simulink model "turbofan"  (R2012b)
settings: Solver=FixedStepDiscrete  StartTime=0.0  StopTime=10.5  FixedStep=0.015  RelTol=1e-3
libraries: Lib_Turbo_Shaft_TMATS x2, Lib_Solve_SSNRSolverJC_TMATS x1
settings Model: Creator=tlavelle  LastModifiedBy=tlavelle

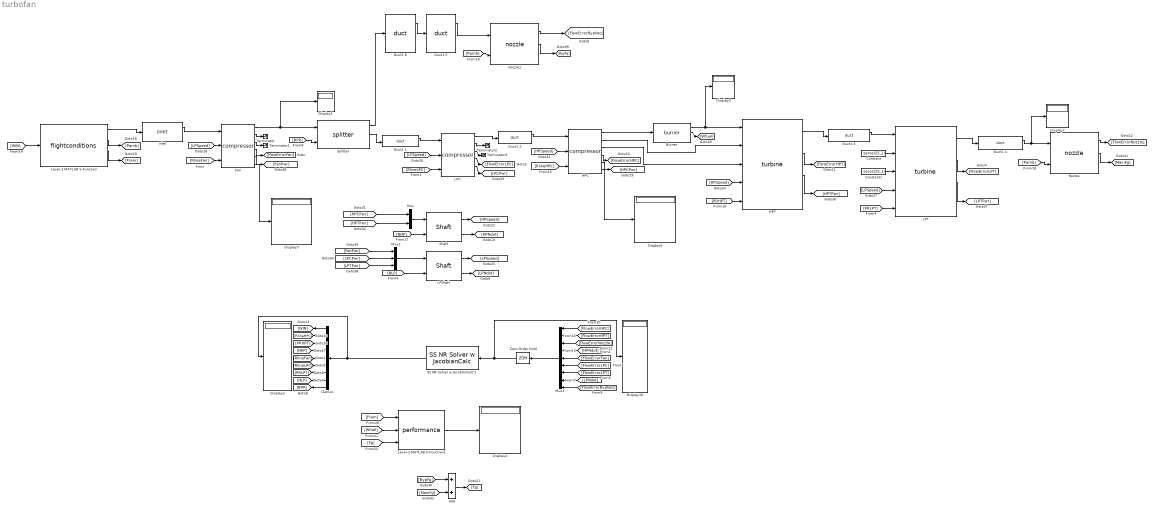
== system turbofan ==
  Add : Sum
  "Burner " : M-S-Function  FunctionName=burner  Parameters=Wfuel,hFuel,dP  mask{Wfuel=.0187, hFuel=-1200, dP=.055}
      mask prompts: Wfuel "FAR"; hFuel "Fuel enthalpy"
      mask Display:
      | color('blue'); port_label('input',1,'Flow In')
      | color('blue'); port_label('output',1,'Flow Out')
      | 
      | color('black'); port_label('output',2,'Wfuel')
  Constant : Constant  Value=zeros(25,1)
  Constant1 : Constant  Value=zeros(25,1)
  Demux : Demux  Outputs=9
  Display{1..7,16} (8 alike) : Display
  Duct1 1 : M-S-Function  FunctionName=duct  Parameters=dP  mask{dP=.0025}
      mask Display:
      | color('blue'); port_label('input',1,'Flow In')
      | color('blue'); port_label('output',1,'Flow Out')
  Duct1 2 : M-S-Function  FunctionName=duct  Parameters=dP  mask{dP=.0025}
      mask Display:
      | color('red'); port_label('input',1,'Flow In')
      | color('red'); port_label('output',1,'Flow Out')
  Duct1 3 : M-S-Function  FunctionName=duct  Parameters=dP  mask{dP=.005}
      mask Display:
      | color('blue'); port_label('input',1,'Flow In')
      | color('blue'); port_label('output',1,'Flow Out')
  Duct1 4 : M-S-Function  FunctionName=duct  Parameters=dP  mask{dP=.01}
      mask Display:
      | color('blue'); port_label('input',1,'Flow In')
      | color('blue'); port_label('output',1,'Flow Out')
  Duct1 5 : M-S-Function  FunctionName=duct  Parameters=dP  mask{dP=.0075}
      mask Display:
      | color('blue'); port_label('input',1,'Flow In')
      | color('blue'); port_label('output',1,'Flow Out')
  Duct1 6 : M-S-Function  FunctionName=duct  Parameters=dP  mask{dP=.0025}
      mask Display:
      | color('blue'); port_label('input',1,'Flow In')
      | color('blue'); port_label('output',1,'Flow Out')
  Fan : M-S-Function  FunctionName=compressor  Parameters=MapFile,NcDes,effDes,PRdes,RlineDes,Wfrac1,hfrac1,Pfrac1,Wfrac2,hfrac2,Pfrac2,s_eff_in,s_PR_in,s_Wc_in,s_C_Nc_in,IDes  mask{MapFile='FAN.map', NcDes=100, effDes=.867, PRdes=1.645, RlineDes=2.3706, Wfrac1=0, hfrac1=0, Pfrac1=0, Wfrac2=0, hfrac2=0, Pfrac2=0, s_eff_in=0, s_PR_in=0, s_Wc_in=0, s_C_Nc_in=0, IDes=0}
      mask prompts: Wfrac1 "Weight Flow Fraction Bleed1"; hfrac1 "Enthalpy Fraction Bleed 1"; Pfrac1 "Pressure Fraction Bleed 1"; Wfrac2 "Weight Flow Fraction Bleed2"; hfrac2 "Enthalpy Fraction Bleed 2"; Pfrac2 "Pressure Fraction 2"; s_eff_in "Efficiency map scalar"; s_PR_in "Pressure ratio map scalar"; s_Wc_in "Corrected weight flow map scalar"; s_C_Nc_in "Corrected speed map scalar"
      mask Display:
      | color('blue'); port_label('input',1,'Flow In')
      | color('red'); port_label('input',2,'Speed')
      | color('darkgreen'); port_label('input',3,'Rline')
      | 
      | color('blue'); port_label('output',1,'Flow Out')
      | color('blue'); port_label('output',2,'Bleed 1')
      | color('blue'); port_label('output',3,'Bleed 2')
      | color('green'); port_label('output',4,'Flow Error')
      | color('black'); port_label('output',5,'Power')
  HPC : M-S-Function  FunctionName=compressor  Parameters=MapFile,NcDes,effDes,PRdes,RlineDes,Wfrac1,hfrac1,Pfrac1,Wfrac2,hfrac2,Pfrac2,s_eff_in,s_PR_in,s_Wc_in,s_C_Nc_in,IDes  mask{MapFile='HPC.map', NcDes=100, effDes=.865, PRdes=5.609, RlineDes=2.0424, Wfrac1=.055, hfrac1=1, Pfrac1=1, Wfrac2=.035, hfrac2=1., Pfrac2=1., s_eff_in=0, s_PR_in=0, s_Wc_in=0, s_C_Nc_in=0, IDes=0}
      mask prompts: Wfrac1 "Weight Flow Fraction Bleed1"; hfrac1 "Enthalpy Fraction Bleed 1"; Pfrac1 "Pressure Fraction Bleed 1"; Wfrac2 "Weight Flow Fraction Bleed2"; hfrac2 "Enthalpy Fraction Bleed 2"; Pfrac2 "Pressure Fraction 2"; s_eff_in "Efficiency map scalar"; s_PR_in "Pressure ratio map scalar"; s_Wc_in "Corrected weight flow map scalar"; s_C_Nc_in "Corrected speed map scalar"
      mask Display:
      | color('blue'); port_label('input',1,'Flow In')
      | color('red'); port_label('input',2,'Speed')
      | color('darkgreen'); port_label('input',3,'Rline')
      | 
      | color('blue'); port_label('output',1,'Flow Out')
      | color('blue'); port_label('output',2,'Bleed 1')
      | color('blue'); port_label('output',3,'Bleed 2')
      | color('green'); port_label('output',4,'Flow Error')
      | color('black'); port_label('output',5,'Power')
  HPT : M-S-Function  FunctionName=turbine  Parameters=MapFile,NcDes,effDes,PRmapDes,Ndes,BSW1,BSW2,s_eff,s_Wc,s_C_Nc,s_PR,IDes  mask{MapFile='HPT1.map', NcDes=100, effDes=.913, PRmapDes=4.9299, Ndes=7499, BSW1=1, BSW2=0, s_eff=0, s_Wc=0, s_C_Nc=0, s_PR=0, IDes=0}
      mask prompts: MapFile "Map File"; NcDes "Design Speed"; effDes "Design efficiency"; PRmapDes "Design Pressure Ratio Map"; Ndes "N des"; BSW1 "Bleed 1 Switch (1 front 0 back)"; BSW2 "Bleed 2 Swtich (1 front 0 back )"; s_eff "Input map efficiency scalar"; s_Wc "Input map correct weight flow scala"; s_C_Nc "Input map speed scalar"; s_PR "Input map pressure ratio scalar"
      mask Display:
      | color('blue'); port_label('input',1,'Flow In')
      | color('blue'); port_label('input',2,'Bleed 1')
      | color('blue'); port_label('input',3,'Bleed 2')
      | color('red'); port_label('input',4,'Speed')
      | color('darkgreen'); port_label('input',5,'PR')
      | 
      | color('blue'); port_label('output',1,'Flow Out')
      | color('green'); port_label('output',2,'Flow Error')
      | color('black'); port_label('output',3,'Power')
  Inlet : M-S-Function  FunctionName=inlet  Parameters=recovery  mask{recovery=.995}
      mask Display:
      | color('blue'); port_label('input',1,'Flow In')
      | color('blue'); port_label('output',1,'Flow Out')
  LPC : M-S-Function  FunctionName=compressor  Parameters=MapFile,NcDes,effDes,PRdes,RlineDes,Wfrac1,hfrac1,Pfrac1,Wfrac2,hfrac2,Pfrac2,s_eff_in,s_PR_in,s_Wc_in,s_C_Nc_in,IDes  mask{MapFile='LPC.map', NcDes=100, effDes=.868, PRdes=2.488, RlineDes=1.7664, Wfrac1=0, hfrac1=0, Pfrac1=0, Wfrac2=0, hfrac2=0, Pfrac2=0, s_eff_in=0, s_PR_in=0, s_Wc_in=0, s_C_Nc_in=0, IDes=0}
      mask prompts: Wfrac1 "Weight Flow Fraction Bleed1"; hfrac1 "Enthalpy Fraction Bleed 1"; Pfrac1 "Pressure Fraction Bleed 1"; Wfrac2 "Weight Flow Fraction Bleed2"; hfrac2 "Enthalpy Fraction Bleed 2"; Pfrac2 "Pressure Fraction 2"; s_eff_in "Efficiency map scalar"; s_PR_in "Pressure ratio map scalar"; s_Wc_in "Corrected weight flow map scalar"
      mask Display:
      | color('blue'); port_label('input',1,'Flow In')
      | color('red'); port_label('input',2,'Speed')
      | color('darkgreen'); port_label('input',3,'Rline')
      | 
      | color('blue'); port_label('output',1,'Flow Out')
      | color('blue'); port_label('output',2,'Bleed 1')
      | color('blue'); port_label('output',3,'Bleed 2')
      | color('green'); port_label('output',4,'Flow Error')
      | color('black'); port_label('output',5,'Power')
  LPShaft : Lib_Turbo_Shaft_TMATS/Shaft  Shaft_Inertia_M=1000
  LPT : M-S-Function  FunctionName=turbine  Parameters=MapFile,NcDes,effDes,PRmapDes,Ndes,BSW1,BSW2,s_eff,s_Wc,s_C_Nc,s_PR,IDes  mask{MapFile='LPT.map', NcDes=100, effDes=.93, PRmapDes=6.4203, Ndes=3723, BSW1=1, BSW2=1, s_eff=0, s_Wc=0, s_C_Nc=0, s_PR=0, IDes=0}
      mask prompts: MapFile "Map File"; NcDes "Design Speed"; effDes "Design efficiency"; PRmapDes "Design Pressure Ratio Map"; Ndes "N des"; BSW1 "Bleed 1 Switch (1 front 0 back)"; BSW2 "Bleed 1 Switch (1 front 0 back)"; s_eff "Input map efficiency scalar"; s_Wc "Input map correct weight flow scalar"; s_C_Nc "Input map speed scalar"; s_PR "Input map pressure ratio scalar"
      mask Display:
      | color('blue'); port_label('input',1,'Flow In')
      | color('blue'); port_label('input',2,'Bleed 1')
      | color('blue'); port_label('input',3,'Bleed 2')
      | color('red'); port_label('input',4,'Speed')
      | color('darkgreen'); port_label('input',5,'PR')
      | 
      | color('blue'); port_label('output',1,'Flow Out')
      | color('green'); port_label('output',2,'Flow Error')
      | color('black'); port_label('output',3,'Power')
  Level-2 MATLAB S-Function : M-S-Function  FunctionName=flightconditions  Parameters=alt,MN,dTs  mask{alt=34000, MN=.8, dTs=0}
      mask prompts: alt "altitude"; MN "Mach Number"; dTs "Ambient Temperature Delta"
      mask Display:
      | color('darkgreen'); port_label('input',1,'Weight Flow')
      | 
      | color('blue'); port_label('output',1,'Flow Out')
      | color('black'); port_label('output',2,'Ambient Pressure')
      | color('black'); port_label('output',3,'Fram')
  Level-2 MATLAB S-Function1 : M-S-Function  FunctionName=performance
      mask Display:
      | color('black'); port_label('input',1,'Fram')
      | color('black'); port_label('input',2,'Wfuel')
      | color('black'); port_label('input',3,'Fg')
      | 
      | color('black'); port_label('output',1,'Performance')
  Mux : Mux  Inputs=2
  Mux1 : Mux  Inputs=9
  Mux2 : Mux  Inputs=3
  Nozzle : M-S-Function  FunctionName=nozzle  Parameters=Wdes,Cfg,Ath_in,IDes  mask{Wdes=113.51, Cfg=.9978, Ath_in=0, IDes=0}
      mask prompts: Wdes "Design Flow"; Ath_in "Throat input area"
      mask Display:
      | color('blue'); port_label('input',1,'Flow In')
      | color('black'); port_label('input',2,'Ambient Pressure')
      | 
      | color('green'); port_label('output',1,'Flow Error')
      | color('black'); port_label('output',2,'Fg')
  Nozzle1 : M-S-Function  FunctionName=nozzle  Parameters=Wdes,Cfg,Ath_in,IDes  mask{Wdes=562.61, Cfg=.9978, Ath_in=0, IDes=0}
      mask prompts: Wdes "Design Flow"; Ath_in "Throat area input"
      mask Display:
      | color('blue'); port_label('input',1,'Flow In')
      | color('black'); port_label('input',2,'Ambient Pressure')
      | 
      | color('green'); port_label('output',1,'Flow Error')
      | color('black'); port_label('output',2,'Fg')
  SS NR Solver w JacobianCalc1 : Lib_Solve_SSNRSolverJC_TMATS/SS NR Solver w JacobianCalc  SJac_Per_M=[1 .01 .01 10 .01 .01 .01 10 .01]  SNR_IC_M=[6742 2 2 7500 2 2 2 4000 5]  SNR_DX_M=10  SJacobianAttempts_M=5  Cond_Limits_M=.1
  Shaft : Lib_Turbo_Shaft_TMATS/Shaft  Shaft_Inertia_M=1000
  "Splitter " : M-S-Function  FunctionName=splitter
      mask Display:
      | color('blue'); port_label('input',1,'Flow In')
      | color('darkgreen'); port_label('input',2,'BPR')
      | 
      | color('blue'); port_label('output',1,'Flow Secondary')
      | color('blue'); port_label('output',2,'Flow Primary')
  Terminator{,1..3} (4 alike) : Terminator
  Zero-Order Hold : ZeroOrderHold  SampleTime=0.015
  wires:
  HPC/1 -> "Burner "/1
  Mux1/1 -> Zero-Order Hold/1
  SS NR Solver w JacobianCalc1/1 -> Display2/1, Demux/1
  "Burner "/1 -> HPT/1, Display3/1
  Shaft/1 -> [HPSpeed]
  "Splitter "/1 -> Duct1 6/1
  Inlet/1 -> Fan/1
  HPT/1 -> Duct1 3/1
  LPT/1 -> Duct1 4/1
  Mux/1 -> Shaft/1
  Mux2/1 -> LPShaft/1
  LPShaft/1 -> [LPSpeed]
  Fan/4 -> [FlowErrorFan]
  [RlineFan] -> Fan/3
  Demux/5 -> [RlineFan]
  [FlowErrorFan] -> Mux1/5
  [RlineLPC] -> LPC/3
  [FlowErrorLPC] -> Mux1/6
  Demux/6 -> [RlineLPC]
  LPT/2 -> [FlowErrorLPT]
  [PRLPT] -> LPT/5
  Demux/7 -> [PRLPT]
  [FlowErrorLPT] -> Mux1/7
  [NLP] -> LPShaft/2
  LPShaft/2 -> [LPNdot]
  [LPNdot] -> Mux1/8
  Demux/8 -> [NLP]
  Demux/9 -> [BPR]
  [FlowErrorBypNoz] -> Mux1/9
  Level-2 MATLAB S-Function/1 -> Inlet/1
  [FlowErrorHPC] -> Mux1/1
  HPC/4 -> [FlowErrorHPC]
  [FlowErrorHPT] -> Mux1/2
  HPT/2 -> [FlowErrorHPT]
  Nozzle/1 -> [FlowErrorNozzle]
  [FlowErrorNozzle] -> Mux1/3
  Shaft/2 -> [HPNdot]
  [HPNdot] -> Mux1/4
  [WIN] -> Level-2 MATLAB S-Function/1
  Demux/1 -> [WIN]
  [RlineHPC] -> HPC/3
  Demux/2 -> [RlineHPC]
  [PRHPT] -> HPT/5
  Demux/3 -> [PRHPT]
  Demux/4 -> [NHP]
  [NHP] -> Shaft/2
  Level-2 MATLAB S-Function/2 -> [Pamb]
  [Pamb] -> Nozzle/2
  Level-2 MATLAB S-Function/3 -> [Fram]
  [BPR] -> "Splitter "/2
  "Burner "/2 -> [Wfuel]
  [MainFg] -> Add/2
  Add/1 -> [Fg]
  [Fram] -> Level-2 MATLAB S-Function1/1
  [Wfuel] -> Level-2 MATLAB S-Function1/2
  [Fg] -> Level-2 MATLAB S-Function1/3
  Level-2 MATLAB S-Function1/1 -> Display4/1
  LPC/4 -> [FlowErrorLPC]
  HPC/3 -> HPT/3
  HPC/2 -> HPT/2
  Fan/1 -> Display1/1, "Splitter "/1
  "Splitter "/2 -> Duct1 1/1
  Duct1 1/1 -> LPC/1
  LPC/1 -> Duct1 2/1
  Duct1 2/1 -> HPC/1
  Duct1 3/1 -> LPT/1
  Duct1 4/1 -> Display7/1, Nozzle/1
  Duct1 6/1 -> Duct1 5/1
  Duct1 5/1 -> Nozzle1/1
  [Pamb] -> Nozzle1/2
  Nozzle1/1 -> [FlowErrorBypNoz]
  [BypFg] -> Add/1
  Fan/2 -> Terminator/1
  Fan/3 -> Terminator1/1
  [HPSpeed] -> HPC/2
  [HPSpeed] -> HPT/4
  [LPSpeed] -> LPC/2
  [LPSpeed] -> LPT/4
  [LPSpeed] -> Fan/2
  LPC/2 -> Terminator2/1
  LPC/3 -> Terminator3/1
  HPT/3 -> [HPTPwr]
  HPC/5 -> [HPCPwr]
  [HPTPwr] -> Mux/2
  [HPCPwr] -> Mux/1
  LPC/5 -> [LPCPwr]
  [LPCPwr] -> Mux2/2
  [FanPwr] -> Mux2/1
  Fan/5 -> [FanPwr]
  LPT/3 -> [LPTPwr]
  [LPTPwr] -> Mux2/3
  Nozzle1/2 -> [BypFg]
  Nozzle/2 -> [MainFg]
  Constant/1 -> LPT/2
  Constant1/1 -> LPT/3
  Zero-Order Hold/1 -> SS NR Solver w JacobianCalc1/1, Display16/1
  Fan/6 -> Display5/1
  HPC/6 -> Display6/1
